simulink model "Q11"  (R2024a)
settings: Solver=FixedStepAuto  StartTime=0.0  StopTime=0.1  FixedStep=1e-5  RelTol=1e-3
undefined symbols (not defined in the file): C, G, H, k, L, P, Ts
settings Model: Creator=psatt  LastModifiedBy=ali
settings RTWCC: GPUComputeCapability=3.5

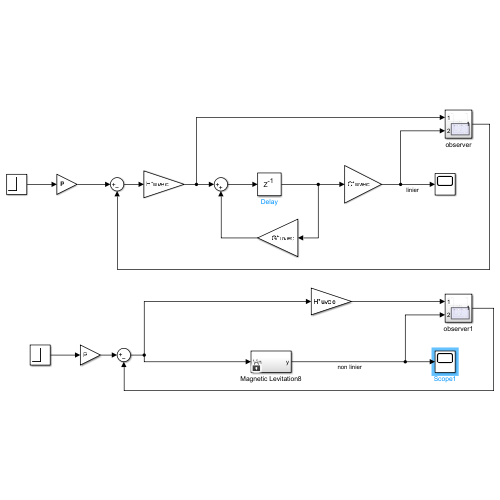
[thumbnail: Simulink's stored preview of the top-level diagram]
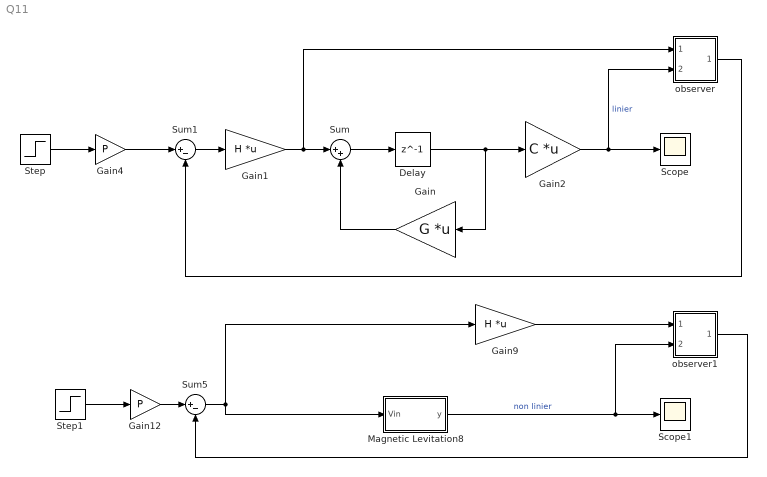
== system Q11 ==
  Delay : Delay  DelayLength=1  SampleTime=Ts
  Gain : Gain  Gain=G  Multiplication=Matrix(K*u) (u vector)
  Gain1 : Gain  Gain=H  Multiplication=Matrix(K*u) (u vector)
  Gain12 : Gain  Gain=P
  Gain2 : Gain  Gain=C  Multiplication=Matrix(K*u) (u vector)
  Gain4 : Gain  Gain=P
  Gain9 : Gain  Gain=H  Multiplication=Matrix(K*u) (u vector)
  Magnetic Levitation8 : Subsystem
  Scope : Scope
  Scope1 : Scope
  Step : Step  Time=0  After=0.002  SampleTime=0
  Step1 : Step  Time=0  After=1e-6  SampleTime=0
  Sum : Sum  Inputs=|++
  Sum1 : Sum  Inputs=|+-
  Sum5 : Sum  Inputs=|+-
  observer : Subsystem
  observer1 : Subsystem
  wires:
  Gain/1 -> Sum/2
  Sum/1 -> Delay/1
  Gain1/1 -> observer/1(In1), Sum/1
  Delay/1 -> Gain/1, Gain2/1
  Sum1/1 -> Gain1/1
  Gain2/1 -> Scope/1, observer/2(In2)  "linier"
  Step/1 -> Gain4/1
  Gain4/1 -> Sum1/1
  Gain12/1 -> Sum5/1
  Step1/1 -> Gain12/1
  Magnetic Levitation8/1(y) -> observer1/2(In2), Scope1/1  "non linier"
  Sum5/1 -> Magnetic Levitation8/1(Vin), Gain9/1
  observer/1(Out1) -> Sum1/2
  Gain9/1 -> observer1/1(In1)
  observer1/1(Out1) -> Sum5/2

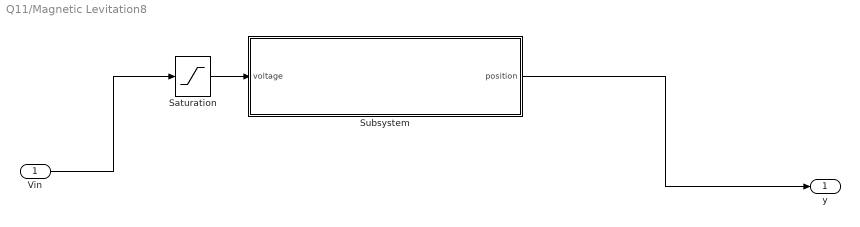
== system Q11/Magnetic Levitation8 ==
  Vin : Inport
  Saturation : Saturate  UpperLimit=10  LowerLimit=-6  ZeroCross=off
  Subsystem : Subsystem
  y : Outport  VectorParamsAs1DForOutWhenUnconnected=off
  wires:
  Vin/1 -> Saturation/1
  Saturation/1 -> Subsystem/1(voltage)
  Subsystem/1("position ") -> y/1

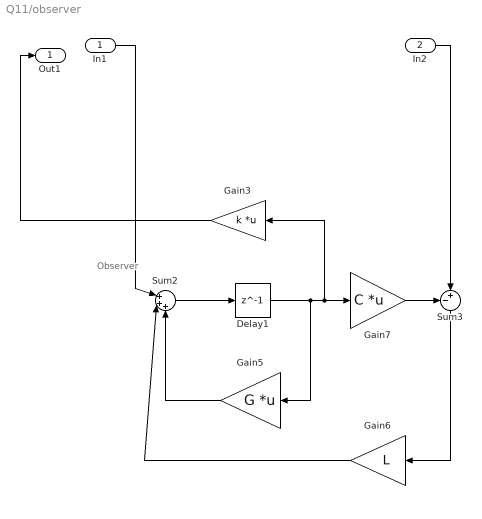
== system Q11/observer ==
  note: Observer
  In1 : Inport
  In2 : Inport  Port=2
  Delay1 : Delay  DelayLength=1  SampleTime=Ts
  Gain3 : Gain  Gain=k  Multiplication=Matrix(K*u) (u vector)
  Gain5 : Gain  Gain=G  Multiplication=Matrix(K*u) (u vector)
  Gain6 : Gain  Gain=L
  Gain7 : Gain  Gain=C  Multiplication=Matrix(K*u) (u vector)
  Sum2 : Sum  Inputs=|+++
  Sum3 : Sum  Inputs=-+|
  Out1 : Outport
  wires:
  Gain7/1 -> Sum3/1
  Delay1/1 -> Gain3/1, Gain7/1, Gain5/1
  Gain5/1 -> Sum2/3
  In1/1 -> Sum2/1
  Sum2/1 -> Delay1/1
  Gain6/1 -> Sum2/2
  Sum3/1 -> Gain6/1
  In2/1 -> Sum3/2
  Gain3/1 -> Out1/1

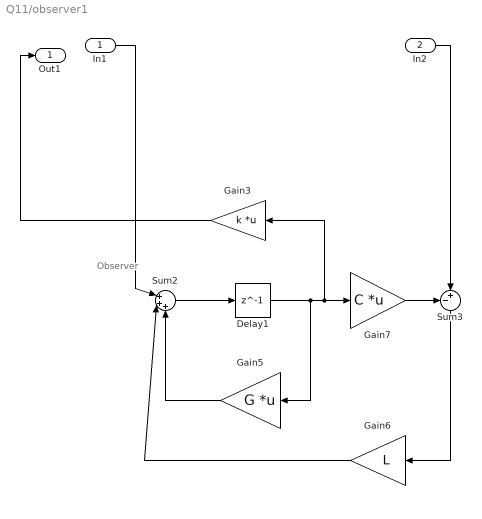
== system Q11/observer1 ==
  note: Observer
  In1 : Inport
  In2 : Inport  Port=2
  Delay1 : Delay  DelayLength=1  SampleTime=Ts
  Gain3 : Gain  Gain=k  Multiplication=Matrix(K*u) (u vector)
  Gain5 : Gain  Gain=G  Multiplication=Matrix(K*u) (u vector)
  Gain6 : Gain  Gain=L
  Gain7 : Gain  Gain=C  Multiplication=Matrix(K*u) (u vector)
  Sum2 : Sum  Inputs=|+++
  Sum3 : Sum  Inputs=-+|
  Out1 : Outport
  wires:
  Gain7/1 -> Sum3/1
  Delay1/1 -> Gain3/1, Gain7/1, Gain5/1
  Gain5/1 -> Sum2/3
  In1/1 -> Sum2/1
  Sum2/1 -> Delay1/1
  Gain6/1 -> Sum2/2
  Sum3/1 -> Gain6/1
  In2/1 -> Sum3/2
  Gain3/1 -> Out1/1

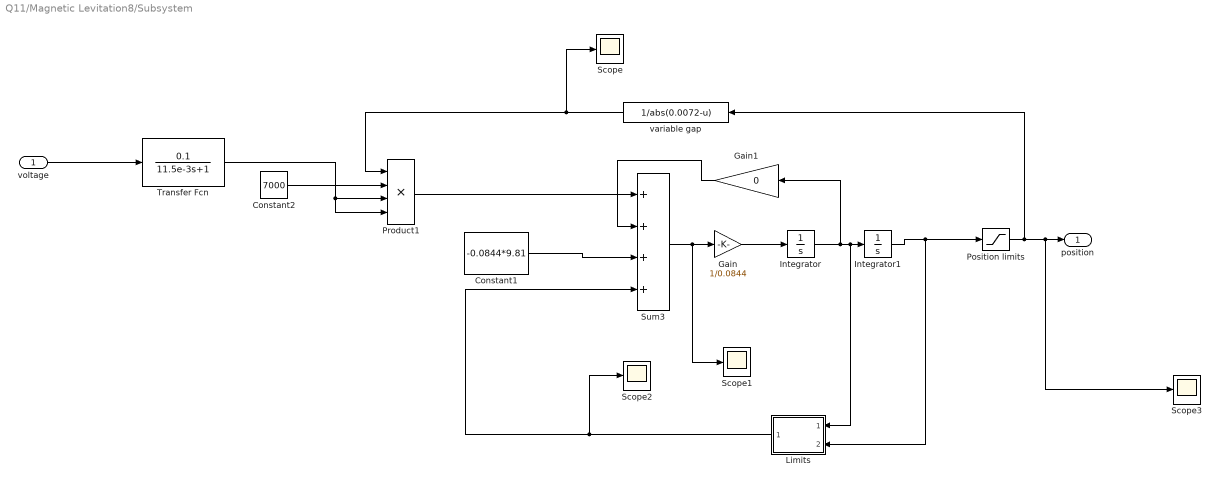
== system Q11/Magnetic Levitation8/Subsystem ==
  voltage : Inport
  Constant1 : Constant  Value=-0.0844*9.81
  Constant2 : Constant  Value=7000
  Gain : Gain  Gain=1/0.0844
  Gain1 : Gain  Gain=0
  Integrator : Integrator
  Integrator1 : Integrator  LimitOutput=on  UpperSaturationLimit=0.005  LowerSaturationLimit=0
  Limits : Subsystem
      mask Display: disp('LIMIT')
  Position limits : Saturate  UpperLimit=0.00499  LowerLimit=0.00001  ZeroCross=off
  Product1 : Product  Inputs=4
  Scope{,1..3} (4 alike) : Scope
  Sum3 : Sum  Inputs=++++
  Transfer Fcn : TransferFcn  Numerator=[0.1]  Denominator=[11.5e-3 1]
  variable gap : Fcn  Expr=1/abs(0.0072-u)
  "position " : Outport  VectorParamsAs1DForOutWhenUnconnected=off
  wires:
  Position limits/1 -> variable gap/1, Scope3/1, "position "/1
  Integrator1/1 -> Limits/2(position), Position limits/1
  Sum3/1 -> Scope1/1, Gain/1
  Constant2/1 -> Product1/2
  Constant1/1 -> Sum3/3
  variable gap/1 -> Scope/1, Product1/1
  Gain1/1 -> Sum3/2
  Gain/1 -> Integrator/1
  Integrator/1 -> Limits/1(velocity), Integrator1/1, Gain1/1
  Product1/1 -> Sum3/1
  Transfer Fcn/1 -> Product1/4, Product1/3
  voltage/1 -> Transfer Fcn/1
  Limits/1(force) -> Scope2/1, Sum3/4

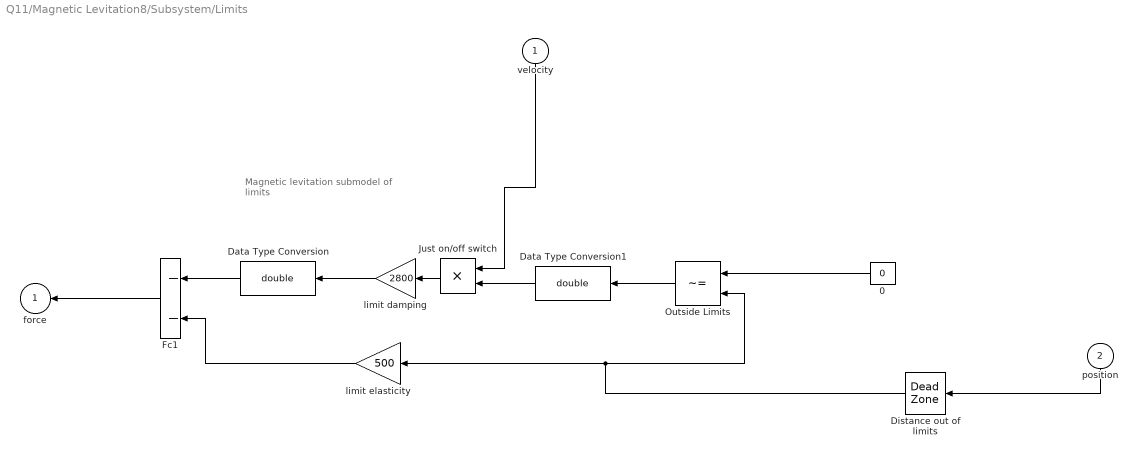
== system Q11/Magnetic Levitation8/Subsystem/Limits ==
  note: Magnetic levitation
      | submodel of limits
  velocity : Inport
  position : Inport  Port=2
  0 : Constant  Value=0
  Data Type Conversion : DataTypeConversion  OutDataTypeStr=double  SaturateOnIntegerOverflow=off  RndMeth=Floor
  Data Type Conversion1 : DataTypeConversion  OutDataTypeStr=double  SaturateOnIntegerOverflow=off  RndMeth=Floor
  Distance out of limits : DeadZone  LowerValue=0.0002  UpperValue=5e-3  ZeroCross=off
  Fc1 : Sum  Inputs=--  InputSameDT=on  SaturateOnIntegerOverflow=on  OutDataTypeStr=Inherit: Same as first input
  "Just on/off switch " : Product  InputSameDT=on  SaturateOnIntegerOverflow=on  OutDataTypeStr=Inherit: Same as first input
  Outside Limits : RelationalOperator  Operator=~=
  limit damping : Gain  Gain=2800  SaturateOnIntegerOverflow=on  OutDataTypeStr=Inherit: Same as input  ParamDataTypeStr=Inherit: Same as input
  limit elasticity : Gain  Gain=500  SaturateOnIntegerOverflow=on  OutDataTypeStr=Inherit: Same as input  ParamDataTypeStr=Inherit: Same as input
  force : Outport  VectorParamsAs1DForOutWhenUnconnected=off
  wires:
  Distance out of limits/1 -> Outside Limits/2, limit elasticity/1
  limit elasticity/1 -> Fc1/2
  Outside Limits/1 -> Data Type Conversion1/1
  0/1 -> Outside Limits/1
  "Just on/off switch "/1 -> limit damping/1
  Fc1/1 -> force/1
  position/1 -> Distance out of limits/1
  limit damping/1 -> Data Type Conversion/1
  Data Type Conversion/1 -> Fc1/1
  velocity/1 -> "Just on/off switch "/1
  Data Type Conversion1/1 -> "Just on/off switch "/2
